simulink model "Green_H2_Solar_Only"  (R2022a)
settings: Solver=daessc  StartTime=0.0  StopTime=3600*3  MaxStep=60/10  RelTol=1e-3  AbsTol=1e-3
undefined symbols (not defined in the file): Control, DH, dT_setpoint, Electric, Plate, R_h2, Solar, TDS
libraries: fl_lib x26, nesl_utility x13, ee_lib x3
(part 4 of 4)

== matlab function Green_H2_Solar_Only/MATLAB Function ==
  data: u input; y output; theta input; dtheta input; Re input
function y = fcn(u, theta, dtheta, Re)
DH = u(1); TDS = u(2);
G0 = DH-((theta-dtheta)/298)*TDS;
y = sqrt(G0*Re);

== matlab function Green_H2_Solar_Only/Sensor/MATLAB Function ==
  data: u input; Z output
function Z = fcn(u)

Z = min(u(2)/u(1),1e3);
